simulink model "validationtool"  (R2021b)
settings: Solver=VariableStepAuto  StartTime=0.0  StopTime=2560  FixedStep=0.5  RelTol=1e-3
StopFcn:
  | msg_bs_ctrl.Data=[0];
  | msg_acc_ctrl.Data=[0 0 0 0 0 0 0 0];
undefined symbols (not defined in the file or in its folder): Battery, canChannel, Ts
libraries: canmsglib x28, canlib x4, sharedTrackingLibrary x1
settings Model: Creator=Roland Kummer  LastModifiedBy=Roland Kummer

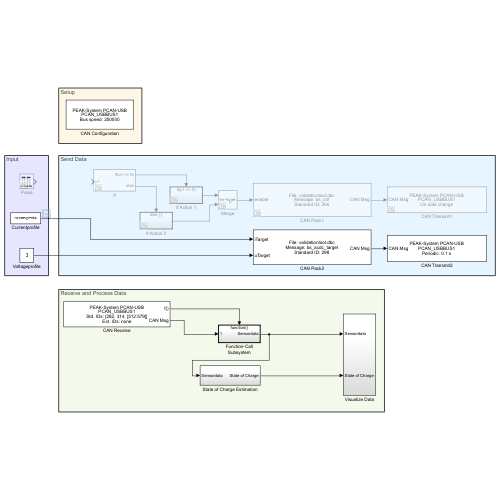
[thumbnail: Simulink's stored preview of the top-level diagram]
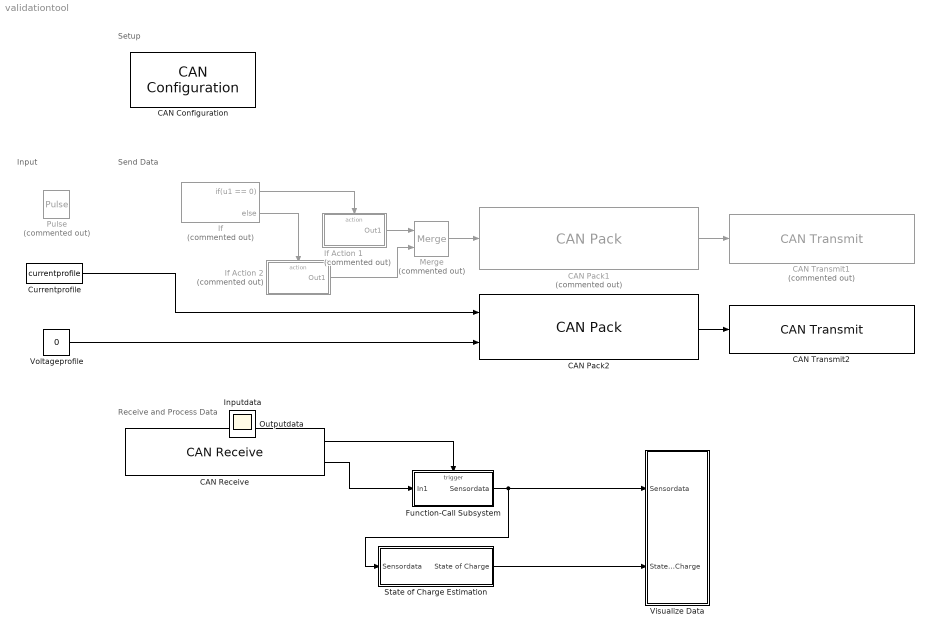
== system validationtool ==
  note: Input
  note: Receive and Process Data
  note: Setup
  note: Send Data
  CAN Configuration : canlib/CAN Configuration  BlockHandle=4.0012  Device=MathWorks Virtual 1 (Channel 1)  DeviceMenu=MathWorks Virtual 1 (Channel 1)  ObjConstructor=canChannel('MathWorks', 'Virtual 1', 1)  BusSpeed=250000  EnableBitParameters=off  AckMode=Normal
      settings: SourceProductBaseCode=VN
  CAN Pack1 : canmsglib/CAN Pack  Commented=on  CANdbFile=C:\Users\Roland Kummer\Documents\Studium\BA-Arbeit\Busmaster\validationtool.dbc  MsgList=bs_ctrl  MsgName=bs_ctrl  MsgIDType=Standard (11-bit identifier)  MsgIdentifier=266  MsgLength=1  Remote=off  ApplyMinMax=off  BusOutput=off  SignalInfo={'enable','0','8','LE','unsigned','Standard','0','1','0','0','2'}
      settings: SourceProductBaseCode=ME,XP,VN  DataFormat=CANdb specified signals
  CAN Pack2 : canmsglib/CAN Pack  CANdbFile=C:\Users\Roland Kummer\Documents\Studium\BA-Arbeit\Busmaster\validationtool.dbc  MsgList=bs_acdc_target  MsgName=bs_acdc_target  MsgIDType=Standard (11-bit identifier)  MsgIdentifier=298  MsgLength=4  Remote=off  ApplyMinMax=off  BusOutput=off  SignalInfo={'iTarget','16','16','LE','unsigned','Standard','0','0.003906','0','0','255.98';'uTarget','0','16','LE','unsigned','Standard','0','0.015625','0','0','0.015625'}
      settings: SourceProductBaseCode=ME,XP,VN  DataFormat=CANdb specified signals
  CAN Receive : canlib/CAN Receive  BlockHandle=7.0012  Device=MathWorks Virtual 1 (Channel 1)  DeviceMenu=MathWorks Virtual 1 (Channel 1)  ObjConstructor=canChannel('MathWorks', 'Virtual 1', 1)  EnableStandardIDsFilter=off  StdIDsCombo=Allow only  StandardIDs=[282, 314, [512:579]]  EnableExtendedIDsFilter=off  ExtIDsCombo=Block all  ExtendedIDs=101  SampleTime=0.1  MsgsPerTimestep=all  InternalFilterUpdateStatus=on  BusOutput=off
      settings: SourceProductBaseCode=VN
  CAN Transmit1 : canlib/CAN Transmit  Commented=on  BlockHandle=8.0012  Device=MathWorks Virtual 1 (Channel 1)  DeviceMenu=MathWorks Virtual 1 (Channel 1)  ObjConstructor=canChannel('MathWorks', 'Virtual 1', 1)  EnableEventTransmit=on  EnablePeriodicTransmit=off  MessagePeriod=0.100
      settings: SourceProductBaseCode=VN
  CAN Transmit2 : canlib/CAN Transmit  BlockHandle=9.0012  Device=MathWorks Virtual 1 (Channel 1)  DeviceMenu=MathWorks Virtual 1 (Channel 1)  ObjConstructor=canChannel('MathWorks', 'Virtual 1', 1)  EnableEventTransmit=off  EnablePeriodicTransmit=on  MessagePeriod=0.100
      settings: SourceProductBaseCode=VN
  Currentprofile : FromWorkspace  VariableName=currentprofile  SampleTime=0.1  Interpolate=off  ZeroCross=off  OutputAfterFinalValue=Setting to zero
  Function-Call Subsystem : Subsystem  TreatAsAtomicUnit=on
  If : If  Commented=on  IfExpression=u1 == 0
  If Action 1 : Subsystem  Commented=on  TreatAsAtomicUnit=on
  If Action 2 : Subsystem  Commented=on  TreatAsAtomicUnit=on
  Merge : Merge  Commented=on
  Pulse : DiscretePulseGenerator  Commented=on  Amplitude=6  Period=1440  PulseWidth=720  PhaseDelay=5
  State of Charge Estimation : Subsystem
  Visualize Data : Subsystem
  Voltageprofile : Constant  Value=0  OutDataTypeStr=double  SampleTime=0.1
  Inputdata : Scope
  Outputdata : Scope
  wires:
  CAN Receive/1 -> Function-Call Subsystem/Trigger
  CAN Receive/2 -> Function-Call Subsystem/1(In1)
  CAN Pack2/1 -> CAN Transmit2/1
  Function-Call Subsystem/1(Sensordata) -> State of Charge Estimation/1(Sensordata), Visualize Data/1(Sensordata)
  State of Charge Estimation/1(State of Charge) -> Visualize Data/2(State of Charge)
  Voltageprofile/1 -> CAN Pack2/2
  CAN Pack1/1 -> CAN Transmit1/1
  If/1 -> If Action 1/Action
  If/2 -> If Action 2/Action
  Merge/1 -> CAN Pack1/1
  If Action 1/1(Out1) -> Merge/1
  If Action 2/1(Out1) -> Merge/2
  Currentprofile/1 -> CAN Pack2/1

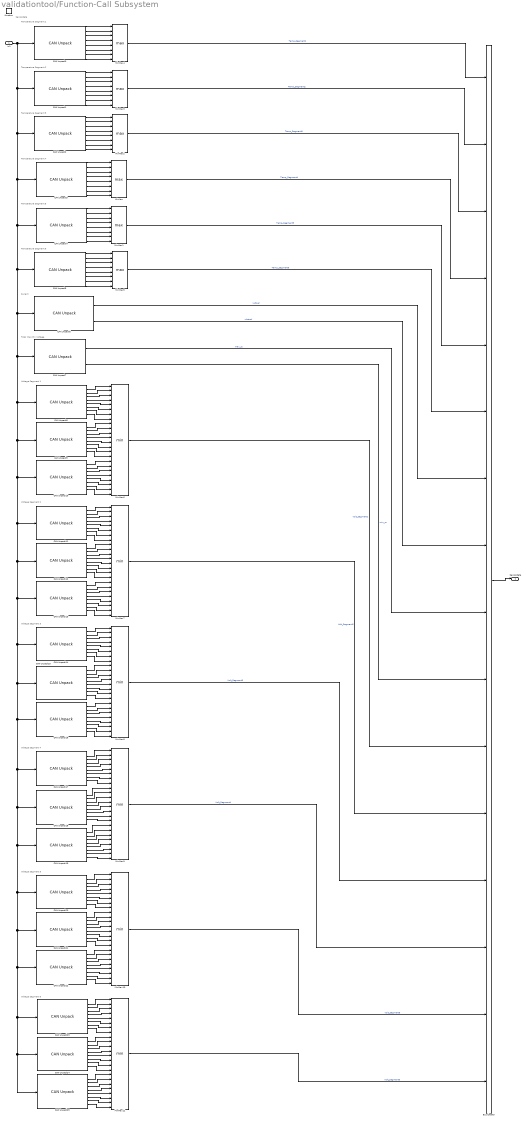
== system validationtool/Function-Call Subsystem ==
  note: Voltage Segment 6
  note: Voltage Segment 2
  note: Voltage Segment 1
  note: Voltage Segment 5
  note: Voltage Segment 4
  note: Voltage Segment 3
  note: Sensordata
  note: Total Max/Min Voltage
  note: Current
  note: Temperature Segment 1
  note: Temperature Segment 2
  note: Temperature Segment 3
  note: Temperature Segment 4
  note: Temperature Segment 6
  note: Temperature Segment 5
  In1 : Inport
  function : TriggerPort  TriggerType=function-call  VariantControl=(inherit)
  Bus Creator : BusCreator  Inputs=16
  CAN Unpack0 : canmsglib/CAN Unpack  CANdbFile=C:\Users\Roland Kummer\Documents\Studium\BA-Arbeit\Busmaster\validationtool.dbc  MsgList=temp1  MsgName=temp1  MsgIDType=Standard (11-bit identifier)  MsgIdentifier=544  MsgLength=8  SignalInfo={'ct1_1','0','8','LE','unsigned','Standard','0','1','0','0','255';'ct1_2','8','8','LE','unsigned','Standard','0','1','0','0','255';'ct1_3','16','8','LE','unsigned','Standard','0','1','0','0','255';'ct1_4','24','8','LE','unsigned','Standard','0','1','0','0','255';'ct1_5','32','8','LE','unsigned','Standard','0','1','0','0','255';'ct1_6','40','8','LE','unsigned','Standard','0','1','0','0','255';'ct1_7','48','8','LE','unsigned','Standard','0','1','0','0','255';'ct1_8','56','1','LE','signed','Standard','0','1','0','0','1'}  IDPort=off  TimestampPort=off  ErrorPort=off  RemotePort=off  LengthPort=off  StatusPort=off  ApplyMinMax=off
      settings: SourceProductBaseCode=ME,XP,VN  DataFormat=CANdb specified signals
  CAN Unpack1 : canmsglib/CAN Unpack  CANdbFile=C:\Users\Roland Kummer\Documents\Studium\BA-Arbeit\Busmaster\validationtool.dbc  MsgList=temp2  MsgName=temp2  MsgIDType=Standard (11-bit identifier)  MsgIdentifier=545  MsgLength=8  SignalInfo={'ct2_1','0','8','LE','unsigned','Standard','0','1','0','0','255';'ct2_2','8','8','LE','unsigned','Standard','0','1','0','0','255';'ct2_3','16','8','LE','unsigned','Standard','0','1','0','0','255';'ct2_4','24','8','LE','unsigned','Standard','0','1','0','0','255';'ct2_5','32','8','LE','unsigned','Standard','0','1','0','0','255';'ct2_6','40','8','LE','unsigned','Standard','0','1','0','0','255';'ct2_7','48','8','LE','unsigned','Standard','0','1','0','0','255';'ct2_8','56','1','LE','signed','Standard','0','1','0','0','1'}  IDPort=off  TimestampPort=off  ErrorPort=off  RemotePort=off  LengthPort=off  StatusPort=off  ApplyMinMax=off
      settings: SourceProductBaseCode=ME,XP,VN  DataFormat=CANdb specified signals
  CAN Unpack10 : canmsglib/CAN Unpack  CANdbFile=C:\Users\Roland Kummer\Documents\Studium\BA-Arbeit\Busmaster\validationtool.dbc  MsgList=cv3  MsgName=cv3  MsgIDType=Standard (11-bit identifier)  MsgIdentifier=514  MsgLength=8  SignalInfo={'cv3_1','0','8','LE','unsigned','Standard','0','0.011765','2','2','5.0001';'cv3_2','8','8','LE','unsigned','Standard','0','0.011765','2','2','5.0001';'cv3_3','16','8','LE','unsigned','Standard','0','0.011765','2','2','5.0001';'cv3_4','24','8','LE','unsigned','Standard','0','0.011765','2','2','5.0001';'cv3_5','32','8','LE','unsigned','Standard','0','0.011765','2','2','5.0001';'cv3_6','40','8','LE','unsigned','Standard','0','0.011765','2','2','5.0001';'cv3_7','48','8','LE','unsigned','Standard','0','0.011765','2','2','5.0001';'cv3_8','56','8','LE','unsigned','Standard','0','0.011765','2','2','5.0001'}  IDPort=off  TimestampPort=off  ErrorPort=off  RemotePort=off  LengthPort=off  StatusPort=off  ApplyMinMax=off
      settings: SourceProductBaseCode=ME,XP,VN  DataFormat=CANdb specified signals
  CAN Unpack11 : canmsglib/CAN Unpack  CANdbFile=C:\Users\Roland Kummer\Documents\Studium\BA-Arbeit\Busmaster\validationtool.dbc  MsgList=cv4  MsgName=cv4  MsgIDType=Standard (11-bit identifier)  MsgIdentifier=515  MsgLength=8  SignalInfo={'cv4_1','0','8','LE','unsigned','Standard','0','0.011765','2','2','5.0001';'cv4_2','8','8','LE','unsigned','Standard','0','0.011765','2','2','5.0001';'cv4_3','16','8','LE','unsigned','Standard','0','0.011765','2','2','5.0001';'cv4_4','24','8','LE','unsigned','Standard','0','0.011765','2','2','5.0001';'cv4_5','32','8','LE','unsigned','Standard','0','0.011765','2','2','5.0001';'cv4_6','40','8','LE','unsigned','Standard','0','0.011765','2','2','5.0001';'cv4_7','48','8','LE','unsigned','Standard','0','0.011765','2','2','5.0001';'cv4_8','56','8','LE','unsigned','Standard','0','0.011765','2','2','5.0001'}  IDPort=off  TimestampPort=off  ErrorPort=off  RemotePort=off  LengthPort=off  StatusPort=off  ApplyMinMax=off
      settings: SourceProductBaseCode=ME,XP,VN  DataFormat=CANdb specified signals
  CAN Unpack12 : canmsglib/CAN Unpack  CANdbFile=C:\Users\Roland Kummer\Documents\Studium\BA-Arbeit\Busmaster\validationtool.dbc  MsgList=cv5  MsgName=cv5  MsgIDType=Standard (11-bit identifier)  MsgIdentifier=516  MsgLength=8  SignalInfo={'cv5_1','0','8','LE','unsigned','Standard','0','0.011765','2','2','5.0001';'cv5_2','8','8','LE','unsigned','Standard','0','0.011765','2','2','5.0001';'cv5_3','16','8','LE','unsigned','Standard','0','0.011765','2','2','5.0001';'cv5_4','24','8','LE','unsigned','Standard','0','0.011765','2','2','5.0001';'cv5_5','32','8','LE','unsigned','Standard','0','0.011765','2','2','5.0001';'cv5_6','40','8','LE','unsigned','Standard','0','0.011765','2','2','5.0001';'cv5_7','48','8','LE','unsigned','Standard','0','0.011765','2','2','5.0001';'cv5_8','56','8','LE','unsigned','Standard','0','0.011765','2','2','5.0001'}  IDPort=off  TimestampPort=off  ErrorPort=off  RemotePort=off  LengthPort=off  StatusPort=off  ApplyMinMax=off
      settings: SourceProductBaseCode=ME,XP,VN  DataFormat=CANdb specified signals
  CAN Unpack13 : canmsglib/CAN Unpack  CANdbFile=C:\Users\Roland Kummer\Documents\Studium\BA-Arbeit\Busmaster\validationtool.dbc  MsgList=cv6  MsgName=cv6  MsgIDType=Standard (11-bit identifier)  MsgIdentifier=517  MsgLength=8  SignalInfo={'cv6_1','0','8','LE','unsigned','Standard','0','0.011765','2','2','5.0001';'cv6_2','8','8','LE','unsigned','Standard','0','0.011765','2','2','5.0001';'cv6_3','16','8','LE','unsigned','Standard','0','0.011765','2','2','5.0001';'cv6_4','24','8','LE','unsigned','Standard','0','0.011765','2','2','5.0001';'cv6_5','32','8','LE','unsigned','Standard','0','0.011765','2','2','5.0001';'cv6_6','40','8','LE','unsigned','Standard','0','0.011765','2','2','5.0001';'cv6_7','48','8','LE','unsigned','Standard','0','0.011765','2','2','5.0001';'cv6_8','56','8','LE','unsigned','Standard','0','0.011765','2','2','5.0001'}  IDPort=off  TimestampPort=off  ErrorPort=off  RemotePort=off  LengthPort=off  StatusPort=off  ApplyMinMax=off
      settings: SourceProductBaseCode=ME,XP,VN  DataFormat=CANdb specified signals
  CAN Unpack14 : canmsglib/CAN Unpack  CANdbFile=C:\Users\Roland Kummer\Documents\Studium\BA-Arbeit\Busmaster\validationtool.dbc  MsgList=cv7  MsgName=cv7  MsgIDType=Standard (11-bit identifier)  MsgIdentifier=518  MsgLength=8  SignalInfo={'cv7_1','0','8','LE','unsigned','Standard','0','0.011765','2','2','5.0001';'cv7_2','8','8','LE','unsigned','Standard','0','0.011765','2','2','5.0001';'cv7_3','16','8','LE','unsigned','Standard','0','0.011765','2','2','5.0001';'cv7_4','24','8','LE','unsigned','Standard','0','0.011765','2','2','5.0001';'cv7_5','32','8','LE','unsigned','Standard','0','0.011765','2','2','5.0001';'cv7_6','40','8','LE','unsigned','Standard','0','0.011765','2','2','5.0001';'cv7_7','48','8','LE','unsigned','Standard','0','0.011765','2','2','5.0001';'cv7_8','56','8','LE','unsigned','Standard','0','0.011765','2','2','5.0001'}  IDPort=off  TimestampPort=off  ErrorPort=off  RemotePort=off  LengthPort=off  StatusPort=off  ApplyMinMax=off
      settings: SourceProductBaseCode=ME,XP,VN  DataFormat=CANdb specified signals
  CAN Unpack15 : canmsglib/CAN Unpack  CANdbFile=C:\Users\Roland Kummer\Documents\Studium\BA-Arbeit\Busmaster\validationtool.dbc  MsgList=cv8  MsgName=cv8  MsgIDType=Standard (11-bit identifier)  MsgIdentifier=519  MsgLength=8  SignalInfo={'cv8_1','0','8','LE','unsigned','Standard','0','0.011765','2','2','5.0001';'cv8_2','8','8','LE','unsigned','Standard','0','0.011765','2','2','5.0001';'cv8_3','16','8','LE','unsigned','Standard','0','0.011765','2','2','5.0001';'cv8_4','24','8','LE','unsigned','Standard','0','0.011765','2','2','5.0001';'cv8_5','32','8','LE','unsigned','Standard','0','0.011765','2','2','5.0001';'cv8_6','40','8','LE','unsigned','Standard','0','0.011765','2','2','5.0001';'cv8_7','48','8','LE','unsigned','Standard','0','0.011765','2','2','5.0001';'cv8_8','56','8','LE','unsigned','Standard','0','0.011765','2','2','5.0001'}  IDPort=off  TimestampPort=off  ErrorPort=off  RemotePort=off  LengthPort=off  StatusPort=off  ApplyMinMax=off
      settings: SourceProductBaseCode=ME,XP,VN  DataFormat=CANdb specified signals
  CAN Unpack16 : canmsglib/CAN Unpack  CANdbFile=C:\Users\Roland Kummer\Documents\Studium\BA-Arbeit\Busmaster\validationtool.dbc  MsgList=cv9  MsgName=cv9  MsgIDType=Standard (11-bit identifier)  MsgIdentifier=520  MsgLength=8  SignalInfo={'cv9_1','0','8','LE','unsigned','Standard','0','0.011765','2','2','5.0001';'cv9_2','8','8','LE','unsigned','Standard','0','0.011765','2','2','5.0001';'cv9_3','16','8','LE','unsigned','Standard','0','0.011765','2','2','5.0001';'cv9_4','24','8','LE','unsigned','Standard','0','0.011765','2','2','5.0001';'cv9_5','32','8','LE','unsigned','Standard','0','0.011765','2','2','5.0001';'cv9_6','40','8','LE','unsigned','Standard','0','0.011765','2','2','5.0001';'cv9_7','48','8','LE','unsigned','Standard','0','0.011765','2','2','5.0001';'cv9_8','56','8','LE','unsigned','Standard','0','0.011765','2','2','5.0001'}  IDPort=off  TimestampPort=off  ErrorPort=off  RemotePort=off  LengthPort=off  StatusPort=off  ApplyMinMax=off
      settings: SourceProductBaseCode=ME,XP,VN  DataFormat=CANdb specified signals
  CAN Unpack17 : canmsglib/CAN Unpack  CANdbFile=C:\Users\Roland Kummer\Documents\Studium\BA-Arbeit\Busmaster\validationtool.dbc  MsgList=cv10  MsgName=cv10  MsgIDType=Standard (11-bit identifier)  MsgIdentifier=521  MsgLength=8  SignalInfo={'cv10_1','0','8','LE','unsigned','Standard','0','0.011765','2','2','5.0001';'cv10_2','8','8','LE','unsigned','Standard','0','0.011765','2','2','5.0001';'cv10_3','16','8','LE','unsigned','Standard','0','0.011765','2','2','5.0001';'cv10_4','24','8','LE','unsigned','Standard','0','0.011765','2','2','5.0001';'cv10_5','32','8','LE','unsigned','Standard','0','0.011765','2','2','5.0001';'cv10_6','40','8','LE','unsigned','Standard','0','0.011765','2','2','5.0001';'cv10_7','48','8','LE','unsigned','Standard','0','0.011765','2','2','5.0001';'cv10_8','56','8','LE','unsigned','Standard','0','0.011765','2','2','5.0001'}  IDPort=off  TimestampPort=off  ErrorPort=off  RemotePort=off  LengthPort=off  StatusPort=off  ApplyMinMax=off
      settings: SourceProductBaseCode=ME,XP,VN  DataFormat=CANdb specified signals
  CAN Unpack18 : canmsglib/CAN Unpack  CANdbFile=C:\Users\Roland Kummer\Documents\Studium\BA-Arbeit\Busmaster\validationtool.dbc  MsgList=cv11  MsgName=cv11  MsgIDType=Standard (11-bit identifier)  MsgIdentifier=522  MsgLength=8  SignalInfo={'cv11_1','0','8','LE','unsigned','Standard','0','0.011765','2','2','5.0001';'cv11_2','8','8','LE','unsigned','Standard','0','0.011765','2','2','5.0001';'cv11_3','16','8','LE','unsigned','Standard','0','0.011765','2','2','5.0001';'cv11_4','24','8','LE','unsigned','Standard','0','0.011765','2','2','5.0001';'cv11_5','32','8','LE','unsigned','Standard','0','0.011765','2','2','5.0001';'cv11_6','40','8','LE','unsigned','Standard','0','0.011765','2','2','5.0001';'cv11_7','48','8','LE','unsigned','Standard','0','0.011765','2','2','5.0001';'cv11_8','56','8','LE','unsigned','Standard','0','0.011765','2','2','5.0001'}  IDPort=off  TimestampPort=off  ErrorPort=off  RemotePort=off  LengthPort=off  StatusPort=off  ApplyMinMax=off
      settings: SourceProductBaseCode=ME,XP,VN  DataFormat=CANdb specified signals
  CAN Unpack19 : canmsglib/CAN Unpack  CANdbFile=C:\Users\Roland Kummer\Documents\Studium\BA-Arbeit\Busmaster\validationtool.dbc  MsgList=cv12  MsgName=cv12  MsgIDType=Standard (11-bit identifier)  MsgIdentifier=523  MsgLength=8  SignalInfo={'cv12_1','0','8','LE','unsigned','Standard','0','0.011765','2','2','5.0001';'cv12_2','8','8','LE','unsigned','Standard','0','0.011765','2','2','5.0001';'cv12_3','16','8','LE','unsigned','Standard','0','0.011765','2','2','5.0001';'cv12_4','24','8','LE','unsigned','Standard','0','0.011765','2','2','5.0001';'cv12_5','32','8','LE','unsigned','Standard','0','0.011765','2','2','5.0001';'cv12_6','40','8','LE','unsigned','Standard','0','0.011765','2','2','5.0001';'cv12_7','48','8','LE','unsigned','Standard','0','0.011765','2','2','5.0001';'cv12_8','56','8','LE','unsigned','Standard','0','0.011765','2','2','5.0001'}  IDPort=off  TimestampPort=off  ErrorPort=off  RemotePort=off  LengthPort=off  StatusPort=off  ApplyMinMax=off
      settings: SourceProductBaseCode=ME,XP,VN  DataFormat=CANdb specified signals
  CAN Unpack2 : canmsglib/CAN Unpack  CANdbFile=C:\Users\Roland Kummer\Documents\Studium\BA-Arbeit\Busmaster\validationtool.dbc  MsgList=temp3  MsgName=temp3  MsgIDType=Standard (11-bit identifier)  MsgIdentifier=546  MsgLength=8  SignalInfo={'ct3_1','0','8','LE','unsigned','Standard','0','1','0','0','255';'ct3_2','8','8','LE','unsigned','Standard','0','1','0','0','255';'ct3_3','16','8','LE','unsigned','Standard','0','1','0','0','255';'ct3_4','24','8','LE','unsigned','Standard','0','1','0','0','255';'ct3_5','32','8','LE','unsigned','Standard','0','1','0','0','255';'ct3_6','40','8','LE','unsigned','Standard','0','1','0','0','255';'ct3_7','48','8','LE','unsigned','Standard','0','1','0','0','255';'ct3_8','56','1','LE','signed','Standard','0','1','0','0','1'}  IDPort=off  TimestampPort=off  ErrorPort=off  RemotePort=off  LengthPort=off  StatusPort=off  ApplyMinMax=off
      settings: SourceProductBaseCode=ME,XP,VN  DataFormat=CANdb specified signals
  CAN Unpack20 : canmsglib/CAN Unpack  CANdbFile=C:\Users\Roland Kummer\Documents\Studium\BA-Arbeit\Busmaster\validationtool.dbc  MsgList=cv13  MsgName=cv13  MsgIDType=Standard (11-bit identifier)  MsgIdentifier=524  MsgLength=8  SignalInfo={'cv13_1','0','8','LE','unsigned','Standard','0','0.011765','2','2','5.0001';'cv13_2','8','8','LE','unsigned','Standard','0','0.011765','2','2','5.0001';'cv13_3','16','8','LE','unsigned','Standard','0','0.011765','2','2','5.0001';'cv13_4','24','8','LE','unsigned','Standard','0','0.011765','2','2','5.0001';'cv13_5','32','8','LE','unsigned','Standard','0','0.011765','2','2','5.0001';'cv13_6','40','8','LE','unsigned','Standard','0','0.011765','2','2','5.0001';'cv13_7','48','8','LE','unsigned','Standard','0','0.011765','2','2','5.0001';'cv13_8','56','8','LE','unsigned','Standard','0','0.011765','2','2','5.0001'}  IDPort=off  TimestampPort=off  ErrorPort=off  RemotePort=off  LengthPort=off  StatusPort=off  ApplyMinMax=off
      settings: SourceProductBaseCode=ME,XP,VN  DataFormat=CANdb specified signals
  CAN Unpack21 : canmsglib/CAN Unpack  CANdbFile=C:\Users\Roland Kummer\Documents\Studium\BA-Arbeit\Busmaster\validationtool.dbc  MsgList=cv14  MsgName=cv14  MsgIDType=Standard (11-bit identifier)  MsgIdentifier=525  MsgLength=8  SignalInfo={'cv14_1','0','8','LE','unsigned','Standard','0','0.011765','2','2','5.0001';'cv14_2','8','8','LE','unsigned','Standard','0','0.011765','2','2','5.0001';'cv14_3','16','8','LE','unsigned','Standard','0','0.011765','2','2','5.0001';'cv14_4','24','8','LE','unsigned','Standard','0','0.011765','2','2','5.0001';'cv14_5','32','8','LE','unsigned','Standard','0','0.011765','2','2','5.0001';'cv14_6','40','8','LE','unsigned','Standard','0','0.011765','2','2','5.0001';'cv14_7','48','8','LE','unsigned','Standard','0','0.011765','2','2','5.0001';'cv14_8','56','8','LE','unsigned','Standard','0','0.011765','2','2','5.0001'}  IDPort=off  TimestampPort=off  ErrorPort=off  RemotePort=off  LengthPort=off  StatusPort=off  ApplyMinMax=off
      settings: SourceProductBaseCode=ME,XP,VN  DataFormat=CANdb specified signals
  CAN Unpack22 : canmsglib/CAN Unpack  CANdbFile=C:\Users\Roland Kummer\Documents\Studium\BA-Arbeit\Busmaster\validationtool.dbc  MsgList=cv15  MsgName=cv15  MsgIDType=Standard (11-bit identifier)  MsgIdentifier=526  MsgLength=8  SignalInfo={'cv15_1','0','8','LE','unsigned','Standard','0','0.011765','2','2','5.0001';'cv15_2','8','8','LE','unsigned','Standard','0','0.011765','2','2','5.0001';'cv15_3','16','8','LE','unsigned','Standard','0','0.011765','2','2','5.0001';'cv15_4','24','8','LE','unsigned','Standard','0','0.011765','2','2','5.0001';'cv15_5','32','8','LE','unsigned','Standard','0','0.011765','2','2','5.0001';'cv15_6','40','8','LE','unsigned','Standard','0','0.011765','2','2','5.0001';'cv15_7','48','8','LE','unsigned','Standard','0','0.011765','2','2','5.0001';'cv15_8','56','8','LE','unsigned','Standard','0','0.011765','2','2','5.0001'}  IDPort=off  TimestampPort=off  ErrorPort=off  RemotePort=off  LengthPort=off  StatusPort=off  ApplyMinMax=off
      settings: SourceProductBaseCode=ME,XP,VN  DataFormat=CANdb specified signals
  CAN Unpack23 : canmsglib/CAN Unpack  CANdbFile=C:\Users\Roland Kummer\Documents\Studium\BA-Arbeit\Busmaster\validationtool.dbc  MsgList=cv16  MsgName=cv16  MsgIDType=Standard (11-bit identifier)  MsgIdentifier=527  MsgLength=8  SignalInfo={'cv16_1','0','8','LE','unsigned','Standard','0','0.011765','2','2','5.0001';'cv16_2','8','8','LE','unsigned','Standard','0','0.011765','2','2','5.0001';'cv16_3','16','8','LE','unsigned','Standard','0','0.011765','2','2','5.0001';'cv16_4','24','8','LE','unsigned','Standard','0','0.011765','2','2','5.0001';'cv16_5','32','8','LE','unsigned','Standard','0','0.011765','2','2','5.0001';'cv16_6','40','8','LE','unsigned','Standard','0','0.011765','2','2','5.0001';'cv16_7','48','8','LE','unsigned','Standard','0','0.011765','2','2','5.0001';'cv16_8','56','8','LE','unsigned','Standard','0','0.011765','2','2','5.0001'}  IDPort=off  TimestampPort=off  ErrorPort=off  RemotePort=off  LengthPort=off  StatusPort=off  ApplyMinMax=off
      settings: SourceProductBaseCode=ME,XP,VN  DataFormat=CANdb specified signals
  CAN Unpack24 : canmsglib/CAN Unpack  CANdbFile=C:\Users\Roland Kummer\Documents\Studium\BA-Arbeit\Busmaster\validationtool.dbc  MsgList=cv17  MsgName=cv17  MsgIDType=Standard (11-bit identifier)  MsgIdentifier=528  MsgLength=8  SignalInfo={'cv17_1','0','8','LE','unsigned','Standard','0','0.011765','2','2','5.0001';'cv17_2','8','8','LE','unsigned','Standard','0','0.011765','2','2','5.0001';'cv17_3','16','8','LE','unsigned','Standard','0','0.011765','2','2','5.0001';'cv17_4','24','8','LE','unsigned','Standard','0','0.011765','2','2','5.0001';'cv17_5','32','8','LE','unsigned','Standard','0','0.011765','2','2','5.0001';'cv17_6','40','8','LE','unsigned','Standard','0','0.011765','2','2','5.0001';'cv17_7','48','8','LE','unsigned','Standard','0','0.011765','2','2','5.0001';'cv17_8','56','8','LE','unsigned','Standard','0','0.011765','2','2','5.0001'}  IDPort=off  TimestampPort=off  ErrorPort=off  RemotePort=off  LengthPort=off  StatusPort=off  ApplyMinMax=off
      settings: SourceProductBaseCode=ME,XP,VN  DataFormat=CANdb specified signals
  CAN Unpack25 : canmsglib/CAN Unpack  CANdbFile=C:\Users\Roland Kummer\Documents\Studium\BA-Arbeit\Busmaster\validationtool.dbc  MsgList=cv18  MsgName=cv18  MsgIDType=Standard (11-bit identifier)  MsgIdentifier=529  MsgLength=8  SignalInfo={'cv18_1','0','8','LE','unsigned','Standard','0','0.011765','2','2','5.0001';'cv18_2','8','8','LE','unsigned','Standard','0','0.011765','2','2','5.0001';'cv18_3','16','8','LE','unsigned','Standard','0','0.011765','2','2','5.0001';'cv18_4','24','8','LE','unsigned','Standard','0','0.011765','2','2','5.0001';'cv18_5','32','8','LE','unsigned','Standard','0','0.011765','2','2','5.0001';'cv18_6','40','8','LE','unsigned','Standard','0','0.011765','2','2','5.0001';'cv18_7','48','8','LE','unsigned','Standard','0','0.011765','2','2','5.0001';'cv18_8','56','8','LE','unsigned','Standard','0','0.011765','2','2','5.0001'}  IDPort=off  TimestampPort=off  ErrorPort=off  RemotePort=off  LengthPort=off  StatusPort=off  ApplyMinMax=off
      settings: SourceProductBaseCode=ME,XP,VN  DataFormat=CANdb specified signals
  CAN Unpack3 : canmsglib/CAN Unpack  CANdbFile=C:\Users\Roland Kummer\Documents\Studium\BA-Arbeit\Busmaster\validationtool.dbc  MsgList=temp4  MsgName=temp4  MsgIDType=Standard (11-bit identifier)  MsgIdentifier=547  MsgLength=8  SignalInfo={'ct4_1','0','8','LE','unsigned','Standard','0','1','0','0','255';'ct4_2','8','8','LE','unsigned','Standard','0','1','0','0','255';'ct4_3','16','8','LE','unsigned','Standard','0','1','0','0','255';'ct4_4','24','8','LE','unsigned','Standard','0','1','0','0','255';'ct4_5','32','8','LE','unsigned','Standard','0','1','0','0','255';'ct4_6','40','8','LE','unsigned','Standard','0','1','0','0','255';'ct4_7','48','8','LE','unsigned','Standard','0','1','0','0','255';'ct4_8','56','1','LE','signed','Standard','0','1','0','0','1'}  IDPort=off  TimestampPort=off  ErrorPort=off  RemotePort=off  LengthPort=off  StatusPort=off  ApplyMinMax=off
      settings: SourceProductBaseCode=ME,XP,VN  DataFormat=CANdb specified signals
  CAN Unpack4 : canmsglib/CAN Unpack  CANdbFile=C:\Users\Roland Kummer\Documents\Studium\BA-Arbeit\Busmaster\validationtool.dbc  MsgList=temp5  MsgName=temp5  MsgIDType=Standard (11-bit identifier)  MsgIdentifier=548  MsgLength=8  SignalInfo={'ct5_1','0','8','LE','unsigned','Standard','0','1','0','0','255';'ct5_2','8','8','LE','unsigned','Standard','0','1','0','0','255';'ct5_3','16','8','LE','unsigned','Standard','0','1','0','0','255';'ct5_4','24','8','LE','unsigned','Standard','0','1','0','0','255';'ct5_5','32','8','LE','unsigned','Standard','0','1','0','0','255';'ct5_6','40','8','LE','unsigned','Standard','0','1','0','0','255';'ct5_7','48','8','LE','unsigned','Standard','0','1','0','0','255';'ct5_8','56','1','LE','signed','Standard','0','1','0','0','1'}  IDPort=off  TimestampPort=off  ErrorPort=off  RemotePort=off  LengthPort=off  StatusPort=off  ApplyMinMax=off
      settings: SourceProductBaseCode=ME,XP,VN  DataFormat=CANdb specified signals
  CAN Unpack5 : canmsglib/CAN Unpack  CANdbFile=C:\Users\Roland Kummer\Documents\Studium\BA-Arbeit\Busmaster\validationtool.dbc  MsgList=temp6  MsgName=temp6  MsgIDType=Standard (11-bit identifier)  MsgIdentifier=549  MsgLength=8  SignalInfo={'ct6_1','0','8','LE','unsigned','Standard','0','1','0','0','255';'ct6_2','8','8','LE','unsigned','Standard','0','1','0','0','255';'ct6_3','16','8','LE','unsigned','Standard','0','1','0','0','255';'ct6_4','24','8','LE','unsigned','Standard','0','1','0','0','255';'ct6_5','32','8','LE','unsigned','Standard','0','1','0','0','255';'ct6_6','40','8','LE','unsigned','Standard','0','1','0','0','255';'ct6_7','48','8','LE','unsigned','Standard','0','1','0','0','255';'ct6_8','56','1','LE','signed','Standard','0','1','0','0','1'}  IDPort=off  TimestampPort=off  ErrorPort=off  RemotePort=off  LengthPort=off  StatusPort=off  ApplyMinMax=off
      settings: SourceProductBaseCode=ME,XP,VN  DataFormat=CANdb specified signals
  CAN Unpack6 : canmsglib/CAN Unpack  CANdbFile=C:\Users\Roland Kummer\Documents\Studium\BA-Arbeit\Busmaster\validationtool.dbc  MsgList=bs_acdc_actual  MsgName=bs_acdc_actual  MsgIDType=Standard (11-bit identifier)  MsgIdentifier=314  MsgLength=4  SignalInfo={'iActual','16','16','LE','unsigned','Standard','0','0.003906','0','0','255.98';'uActual','0','16','LE','unsigned','Standard','0','0.015625','0','0','1023.98'}  IDPort=off  TimestampPort=off  ErrorPort=off  RemotePort=off  LengthPort=off  StatusPort=off  ApplyMinMax=off
      settings: SourceProductBaseCode=ME,XP,VN  DataFormat=CANdb specified signals
  CAN Unpack7 : canmsglib/CAN Unpack  CANdbFile=C:\Users\Roland Kummer\Documents\Studium\BA-Arbeit\Busmaster\validationtool.dbc  MsgList=accu_signal_1  MsgName=accu_signal_1  MsgIDType=Standard (11-bit identifier)  MsgIdentifier=576  MsgLength=8  SignalInfo={'max_cv','8','16','BE','unsigned','Standard','0','0.0001','0','0','6.5535';'min_cv','24','16','BE','unsigned','Standard','0','0.0001','0','0','6.5535'}  IDPort=off  TimestampPort=off  ErrorPort=off  RemotePort=off  LengthPort=off  StatusPort=off  ApplyMinMax=off
      settings: SourceProductBaseCode=ME,XP,VN  DataFormat=CANdb specified signals
  CAN Unpack8 : canmsglib/CAN Unpack  CANdbFile=C:\Users\Roland Kummer\Documents\Studium\BA-Arbeit\Busmaster\validationtool.dbc  MsgList=cv1  MsgName=cv1  MsgIDType=Standard (11-bit identifier)  MsgIdentifier=512  MsgLength=8  SignalInfo={'cv1_1','0','8','LE','unsigned','Standard','0','0.011765','2','2','5.0001';'cv1_2','8','8','LE','unsigned','Standard','0','0.011765','2','2','5.0001';'cv1_3','16','8','LE','unsigned','Standard','0','0.011765','2','2','5.0001';'cv1_4','24','8','LE','unsigned','Standard','0','0.011765','2','2','5.0001';'cv1_5','32','8','LE','unsigned','Standard','0','0.011765','2','2','5.0001';'cv1_6','40','8','LE','unsigned','Standard','0','0.011765','2','2','5.0001';'cv1_7','48','8','LE','unsigned','Standard','0','0.011765','2','2','5.0001';'cv1_8','56','8','LE','unsigned','Standard','0','0.011765','2','2','5.0001'}  IDPort=off  TimestampPort=off  ErrorPort=off  RemotePort=off  LengthPort=off  StatusPort=off  ApplyMinMax=off
      settings: SourceProductBaseCode=ME,XP,VN  DataFormat=CANdb specified signals
  CAN Unpack9 : canmsglib/CAN Unpack  CANdbFile=C:\Users\Roland Kummer\Documents\Studium\BA-Arbeit\Busmaster\validationtool.dbc  MsgList=cv2  MsgName=cv2  MsgIDType=Standard (11-bit identifier)  MsgIdentifier=513  MsgLength=8  SignalInfo={'cv2_1','0','8','LE','unsigned','Standard','0','0.011765','2','2','5.0001';'cv2_2','8','8','LE','unsigned','Standard','0','0.011765','2','2','5.0001';'cv2_3','16','8','LE','unsigned','Standard','0','0.011765','2','2','5.0001';'cv2_4','24','8','LE','unsigned','Standard','0','0.011765','2','2','5.0001';'cv2_5','32','8','LE','unsigned','Standard','0','0.011765','2','2','5.0001';'cv2_6','40','8','LE','unsigned','Standard','0','0.011765','2','2','5.0001';'cv2_7','48','8','LE','unsigned','Standard','0','0.011765','2','2','5.0001';'cv2_8','56','8','LE','unsigned','Standard','0','0.011765','2','2','5.0001'}  IDPort=off  TimestampPort=off  ErrorPort=off  RemotePort=off  LengthPort=off  StatusPort=off  ApplyMinMax=off
      settings: SourceProductBaseCode=ME,XP,VN  DataFormat=CANdb specified signals
  MinMax{,1..5} (6 alike) : MinMax  Function=max  Inputs=8
  MinMax{6..11} (6 alike) : MinMax  Inputs=24
  Sensordata : Outport
  wires:
  In1/1 -> CAN Unpack6/1, CAN Unpack7/1, CAN Unpack8/1, CAN Unpack9/1, CAN Unpack10/1, CAN Unpack11/1, CAN Unpack12/1, CAN Unpack13/1, CAN Unpack14/1, CAN Unpack15/1, CAN Unpack16/1, CAN Unpack17/1, CAN Unpack18/1, CAN Unpack19/1, CAN Unpack20/1, CAN Unpack21/1, CAN Unpack22/1, CAN Unpack23/1, CAN Unpack24/1, CAN Unpack25/1, CAN Unpack5/1, CAN Unpack4/1, CAN Unpack3/1, CAN Unpack2/1, CAN Unpack1/1, CAN Unpack0/1
  CAN Unpack13/8 -> MinMax7/24
  CAN Unpack8/1 -> MinMax6/1
  CAN Unpack8/2 -> MinMax6/2
  CAN Unpack8/3 -> MinMax6/3
  CAN Unpack8/5 -> MinMax6/5
  CAN Unpack8/6 -> MinMax6/6
  CAN Unpack8/7 -> MinMax6/7
  CAN Unpack8/8 -> MinMax6/8
  CAN Unpack9/1 -> MinMax6/9
  CAN Unpack9/2 -> MinMax6/10
  CAN Unpack9/3 -> MinMax6/11
  CAN Unpack9/4 -> MinMax6/12
  CAN Unpack9/5 -> MinMax6/13
  CAN Unpack9/6 -> MinMax6/14
  CAN Unpack9/7 -> MinMax6/15
  CAN Unpack9/8 -> MinMax6/16
  CAN Unpack10/1 -> MinMax6/17
  CAN Unpack10/2 -> MinMax6/18
  CAN Unpack10/3 -> MinMax6/19
  CAN Unpack10/4 -> MinMax6/20
  CAN Unpack10/5 -> MinMax6/21
  CAN Unpack10/6 -> MinMax6/22
  CAN Unpack10/7 -> MinMax6/23
  CAN Unpack10/8 -> MinMax6/24
  CAN Unpack11/1 -> MinMax7/1
  CAN Unpack11/2 -> MinMax7/2
  CAN Unpack11/3 -> MinMax7/3
  CAN Unpack11/4 -> MinMax7/4
  CAN Unpack11/5 -> MinMax7/5
  CAN Unpack11/6 -> MinMax7/6
  CAN Unpack11/7 -> MinMax7/7
  CAN Unpack11/8 -> MinMax7/8
  CAN Unpack12/1 -> MinMax7/9
  CAN Unpack12/2 -> MinMax7/10
  CAN Unpack12/3 -> MinMax7/11
  CAN Unpack12/4 -> MinMax7/12
  CAN Unpack12/5 -> MinMax7/13
  CAN Unpack12/6 -> MinMax7/14
  CAN Unpack12/7 -> MinMax7/15
  CAN Unpack12/8 -> MinMax7/16
  CAN Unpack13/1 -> MinMax7/17
  CAN Unpack13/2 -> MinMax7/18
  CAN Unpack13/3 -> MinMax7/19
  CAN Unpack13/4 -> MinMax7/20
  CAN Unpack13/5 -> MinMax7/21
  CAN Unpack13/6 -> MinMax7/22
  CAN Unpack13/7 -> MinMax7/23
  CAN Unpack14/1 -> MinMax8/1
  CAN Unpack14/2 -> MinMax8/2
  CAN Unpack14/3 -> MinMax8/3
  CAN Unpack14/4 -> MinMax8/4
  CAN Unpack14/5 -> MinMax8/5
  CAN Unpack14/6 -> MinMax8/6
  CAN Unpack14/7 -> MinMax8/7
  CAN Unpack14/8 -> MinMax8/8
  CAN Unpack15/1 -> MinMax8/9
  CAN Unpack15/2 -> MinMax8/10
  CAN Unpack15/3 -> MinMax8/11
  CAN Unpack15/4 -> MinMax8/12
  CAN Unpack15/5 -> MinMax8/13
  CAN Unpack15/6 -> MinMax8/14
  CAN Unpack15/7 -> MinMax8/15
  CAN Unpack15/8 -> MinMax8/16
  CAN Unpack16/1 -> MinMax8/17
  CAN Unpack16/2 -> MinMax8/18
  CAN Unpack16/3 -> MinMax8/19
  CAN Unpack16/4 -> MinMax8/20
  CAN Unpack16/5 -> MinMax8/21
  CAN Unpack16/6 -> MinMax8/22
  CAN Unpack16/7 -> MinMax8/23
  CAN Unpack16/8 -> MinMax8/24
  CAN Unpack17/1 -> MinMax9/1
  CAN Unpack17/2 -> MinMax9/2
  CAN Unpack17/3 -> MinMax9/3
  CAN Unpack17/4 -> MinMax9/4
  CAN Unpack17/5 -> MinMax9/5
  CAN Unpack17/6 -> MinMax9/6
  CAN Unpack17/7 -> MinMax9/7
  CAN Unpack17/8 -> MinMax9/8
  CAN Unpack18/1 -> MinMax9/9
  CAN Unpack18/2 -> MinMax9/10
  CAN Unpack18/3 -> MinMax9/11
  CAN Unpack18/4 -> MinMax9/12
  CAN Unpack18/5 -> MinMax9/13
  CAN Unpack18/6 -> MinMax9/14
  CAN Unpack18/7 -> MinMax9/15
  CAN Unpack18/8 -> MinMax9/16
  CAN Unpack19/1 -> MinMax9/17
  CAN Unpack19/2 -> MinMax9/18
  CAN Unpack19/3 -> MinMax9/19
  CAN Unpack19/4 -> MinMax9/20
  CAN Unpack19/5 -> MinMax9/21
  CAN Unpack19/6 -> MinMax9/22
  CAN Unpack19/7 -> MinMax9/23
  CAN Unpack19/8 -> MinMax9/24
  CAN Unpack20/1 -> MinMax10/1
  CAN Unpack20/2 -> MinMax10/2
  CAN Unpack20/3 -> MinMax10/3
  CAN Unpack20/4 -> MinMax10/4
  CAN Unpack20/5 -> MinMax10/5
  CAN Unpack20/6 -> MinMax10/6
  CAN Unpack20/7 -> MinMax10/7
  CAN Unpack20/8 -> MinMax10/8
  CAN Unpack21/1 -> MinMax10/9
  CAN Unpack21/2 -> MinMax10/10
  CAN Unpack21/3 -> MinMax10/11
  CAN Unpack21/4 -> MinMax10/12
  CAN Unpack21/5 -> MinMax10/13
  CAN Unpack21/6 -> MinMax10/14
  CAN Unpack21/7 -> MinMax10/15
  CAN Unpack21/8 -> MinMax10/16
  CAN Unpack22/1 -> MinMax10/17
  CAN Unpack22/2 -> MinMax10/18
  CAN Unpack22/3 -> MinMax10/19
  CAN Unpack22/4 -> MinMax10/20
  CAN Unpack22/5 -> MinMax10/21
  CAN Unpack22/6 -> MinMax10/22
  CAN Unpack22/7 -> MinMax10/23
  CAN Unpack22/8 -> MinMax10/24
  CAN Unpack23/1 -> MinMax11/1
  CAN Unpack23/2 -> MinMax11/2
  CAN Unpack23/3 -> MinMax11/3
  CAN Unpack23/4 -> MinMax11/4
  CAN Unpack23/5 -> MinMax11/5
  CAN Unpack23/6 -> MinMax11/6
  CAN Unpack23/7 -> MinMax11/7
  CAN Unpack23/8 -> MinMax11/8
  CAN Unpack24/1 -> MinMax11/9
  CAN Unpack24/2 -> MinMax11/10
  CAN Unpack24/3 -> MinMax11/11
  CAN Unpack24/4 -> MinMax11/12
  CAN Unpack24/5 -> MinMax11/13
  CAN Unpack24/6 -> MinMax11/14
  CAN Unpack24/7 -> MinMax11/15
  CAN Unpack24/8 -> MinMax11/16
  CAN Unpack25/1 -> MinMax11/17
  CAN Unpack25/2 -> MinMax11/18
  CAN Unpack25/3 -> MinMax11/19
  CAN Unpack25/4 -> MinMax11/20
  CAN Unpack25/5 -> MinMax11/21
  CAN Unpack25/6 -> MinMax11/22
  CAN Unpack25/7 -> MinMax11/23
  CAN Unpack25/8 -> MinMax11/24
  MinMax4/1 -> Bus Creator/1  "Temp_Segment1"
  MinMax3/1 -> Bus Creator/2  "Temp_Segment2"
  MinMax2/1 -> Bus Creator/3  "Temp_Segment3"
  MinMax/1 -> Bus Creator/4  "Temp_Segment4"
  MinMax5/1 -> Bus Creator/6  "Temp_Segment6"
  CAN Unpack7/1 -> Bus Creator/9  "max_cv"
  CAN Unpack7/2 -> Bus Creator/10  "min_cv"
  MinMax1/1 -> Bus Creator/5  "Temp_Segment5"
  Bus Creator/1 -> Sensordata/1
  MinMax6/1 -> Bus Creator/11  "Volt_Segment1"
  MinMax7/1 -> Bus Creator/12  "Volt_Segment2"
  MinMax8/1 -> Bus Creator/13  "Volt_Segment3"
  MinMax9/1 -> Bus Creator/14  "Volt_Segment4"
  MinMax10/1 -> Bus Creator/15  "Volt_Segment5"
  MinMax11/1 -> Bus Creator/16  "Volt_Segment6"
  CAN Unpack6/1 -> Bus Creator/7  "iActual"
  CAN Unpack6/2 -> Bus Creator/8  "uActual"
  CAN Unpack8/4 -> MinMax6/4
  CAN Unpack0/1 -> MinMax4/1
  CAN Unpack0/2 -> MinMax4/2
  CAN Unpack0/3 -> MinMax4/3
  CAN Unpack0/4 -> MinMax4/4
  CAN Unpack0/5 -> MinMax4/5
  CAN Unpack0/6 -> MinMax4/6
  CAN Unpack0/7 -> MinMax4/7
  CAN Unpack0/8 -> MinMax4/8
  CAN Unpack1/1 -> MinMax3/1
  CAN Unpack1/2 -> MinMax3/2
  CAN Unpack1/3 -> MinMax3/3
  CAN Unpack1/4 -> MinMax3/4
  CAN Unpack1/5 -> MinMax3/5
  CAN Unpack1/6 -> MinMax3/6
  CAN Unpack1/7 -> MinMax3/7
  CAN Unpack1/8 -> MinMax3/8
  CAN Unpack2/1 -> MinMax2/1
  CAN Unpack2/2 -> MinMax2/2
  CAN Unpack2/3 -> MinMax2/3
  CAN Unpack2/4 -> MinMax2/4
  CAN Unpack2/5 -> MinMax2/5
  CAN Unpack2/6 -> MinMax2/6
  CAN Unpack2/7 -> MinMax2/7
  CAN Unpack2/8 -> MinMax2/8
  CAN Unpack3/1 -> MinMax/1
  CAN Unpack3/2 -> MinMax/2
  CAN Unpack3/3 -> MinMax/3
  CAN Unpack3/4 -> MinMax/4
  CAN Unpack3/5 -> MinMax/5
  CAN Unpack3/6 -> MinMax/6
  CAN Unpack3/7 -> MinMax/7
  CAN Unpack3/8 -> MinMax/8
  CAN Unpack4/1 -> MinMax1/1
  CAN Unpack4/2 -> MinMax1/2
  CAN Unpack4/3 -> MinMax1/3
  CAN Unpack4/4 -> MinMax1/4
  CAN Unpack4/5 -> MinMax1/5
  CAN Unpack4/6 -> MinMax1/6
  CAN Unpack4/7 -> MinMax1/7
  CAN Unpack4/8 -> MinMax1/8
  CAN Unpack5/1 -> MinMax5/1
  CAN Unpack5/2 -> MinMax5/2
  CAN Unpack5/3 -> MinMax5/3
  CAN Unpack5/4 -> MinMax5/4
  CAN Unpack5/5 -> MinMax5/5
  CAN Unpack5/6 -> MinMax5/6
  CAN Unpack5/7 -> MinMax5/7
  CAN Unpack5/8 -> MinMax5/8

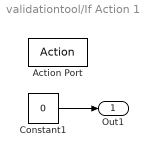
== system validationtool/If Action 1 ==
  Action Port : ActionPort  ActionPortLabel=if(u1 == 0)
  Constant1 : Constant  Value=0  OutDataTypeStr=double  SampleTime=1
  Out1 : Outport
  wires:
  Constant1/1 -> Out1/1

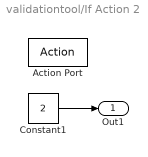
== system validationtool/If Action 2 ==
  Action Port : ActionPort  ActionPortLabel=else
  Constant1 : Constant  Value=2  OutDataTypeStr=double  SampleTime=1
  Out1 : Outport
  wires:
  Constant1/1 -> Out1/1

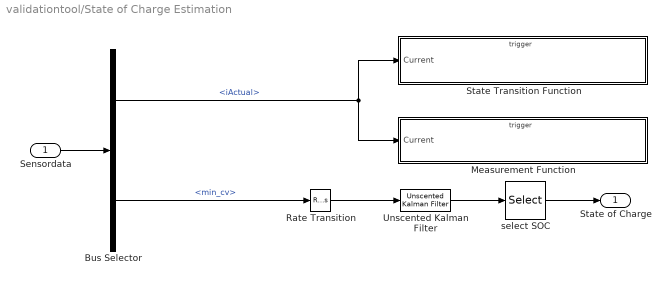
== system validationtool/State of Charge Estimation ==
  Sensordata : Inport
  Bus Selector : BusSelector  OutputSignals=iActual,min_cv
  Measurement Function : Subsystem  TreatAsAtomicUnit=on
  Rate Transition : RateTransition
  State Transition Function : Subsystem  TreatAsAtomicUnit=on
  Unscented Kalman Filter : sharedTrackingLibrary/Unscented Kalman Filter  StateTransitionFcn=StateFcn  HasAdditiveProcessNoise=Additive  ProcessNoise=1e-10*eye(3)  HasTimeVaryingProcessNoise=off  HasStateTransitionFcnExtraArgument=0  InitialState=[0.95; 0; 0]  InitialStateCovariance=[1e-2 1 1]  Alpha=1  Beta=2  Kappa=0  MeasurementFcn1=MeasurementFcn  HasMeasurementEnablePort1=off  HasAdditiveMeasurementNoise1=Additive  MeasurementNoise1=0.5  HasTimeVaryingMeasurementNoise1=off  HasMeasurementFcnExtraArgument1=0  MeasurementFcn2=myMeasurementFcn  HasMeasurementEnablePort2=off  HasAdditiveMeasurementNoise2=Additive  MeasurementNoise2=1  HasTimeVaryingMeasurementNoise2=off  HasMeasurementFcnExtraArgument2=0  MeasurementFcn3=myMeasurementFcn  HasMeasurementEnablePort3=off  HasAdditiveMeasurementNoise3=Additive  MeasurementNoise3=1  HasTimeVaryingMeasurementNoise3=off  HasMeasurementFcnExtraArgument3=0  MeasurementFcn4=myMeasurementFcn  HasMeasurementEnablePort4=off  HasAdditiveMeasurementNoise4=Additive  MeasurementNoise4=1  HasTimeVaryingMeasurementNoise4=off  HasMeasurementFcnExtraArgument4=0  MeasurementFcn5=myMeasurementFcn  HasMeasurementEnablePort5=off  HasAdditiveMeasurementNoise5=Additive  MeasurementNoise5=1  HasTimeVaryingMeasurementNoise5=off  HasMeasurementFcnExtraArgument5=0  EnableMultirate=off  StateTransitionFcnSampleTime=-1  MeasurementFcn1SampleTime=-1  MeasurementFcn2SampleTime=-1  MeasurementFcn3SampleTime=-1  MeasurementFcn4SampleTime=-1  MeasurementFcn5SampleTime=-1  UseCurrentEstimator=on  OutputStateCovariance=off  DataType=double  SampleTime=Ts  NumberOfMeasurements=1
      settings: SourceProductBaseCode=CT
  select SOC : Selector  InputPortWidth=3  IndexOptions=Index vector (dialog)  Indices=1  OutputSizes=1
  State of Charge : Outport
  wires:
  Sensordata/1 -> Bus Selector/1
  Bus Selector/2 -> Rate Transition/1  "<min_cv>"
  Bus Selector/1 -> State Transition Function/1(Current), Measurement Function/1(Current)  "<iActual>"
  Unscented Kalman Filter/1 -> select SOC/1
  Rate Transition/1 -> Unscented Kalman Filter/1
  select SOC/1 -> State of Charge/1

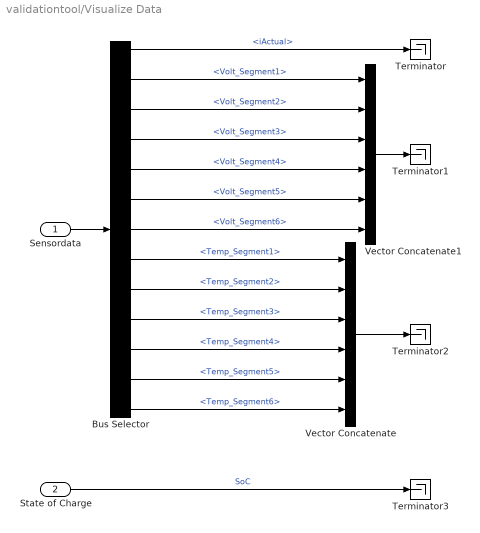
== system validationtool/Visualize Data ==
  Sensordata : Inport
  State of Charge : Inport  Port=2
  Bus Selector : BusSelector  OutputSignals=iActual,Volt_Segment1,Volt_Segment2,Volt_Segment3,Volt_Segment4,Volt_Segment5,Volt_Segment6,Temp_Segment1,Temp_Segment2,Temp_Segment3,Temp_Segment4,Temp_Segment5,Temp_Segment6
  Terminator{,1..3} (4 alike) : Terminator
  Vector Concatenate : Concatenate  NumInputs=6
  Vector Concatenate1 : Concatenate  NumInputs=6
  wires:
  Sensordata/1 -> Bus Selector/1
  Bus Selector/8 -> Vector Concatenate/1  "<Temp_Segment1>"
  Bus Selector/9 -> Vector Concatenate/2  "<Temp_Segment2>"
  Bus Selector/10 -> Vector Concatenate/3  "<Temp_Segment3>"
  Bus Selector/11 -> Vector Concatenate/4  "<Temp_Segment4>"
  Bus Selector/12 -> Vector Concatenate/5  "<Temp_Segment5>"
  Bus Selector/13 -> Vector Concatenate/6  "<Temp_Segment6>"
  Vector Concatenate/1 -> Terminator2/1
  Bus Selector/2 -> Vector Concatenate1/1  "<Volt_Segment1>"
  Bus Selector/3 -> Vector Concatenate1/2  "<Volt_Segment2>"
  Bus Selector/4 -> Vector Concatenate1/3  "<Volt_Segment3>"
  Bus Selector/5 -> Vector Concatenate1/4  "<Volt_Segment4>"
  Bus Selector/6 -> Vector Concatenate1/5  "<Volt_Segment5>"
  Bus Selector/7 -> Vector Concatenate1/6  "<Volt_Segment6>"
  Vector Concatenate1/1 -> Terminator1/1
  Bus Selector/1 -> Terminator/1  "<iActual>"
  State of Charge/1 -> Terminator3/1  "SoC"

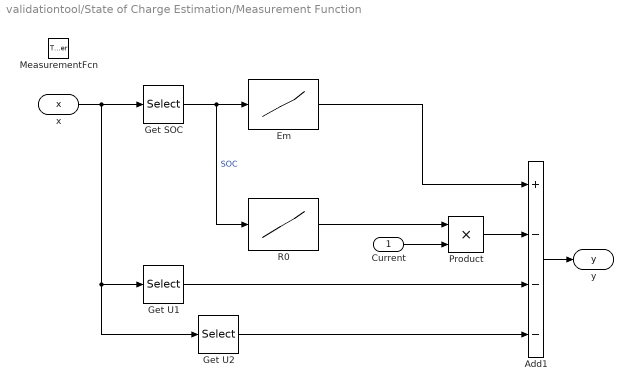
== system validationtool/State of Charge Estimation/Measurement Function ==
  Current : Inport
  MeasurementFcn : TriggerPort  TriggerType=function-call  IsSimulinkFunction=on  FunctionName=MeasurementFcn  VariantControl=Variant
  Add1 : Sum  Inputs=+---
  Em : Lookup_n-D  NumberOfTableDimensions=1  BreakpointsForDimension1=Battery.SOC_LUT  BreakpointsForDimension2=Battery.Temperature_LUT  Table=Battery.Em_LUT  InternalRulePriority=Speed  RndMeth=Simplest  InputSameDT=on
  Get SOC : Selector  InputPortWidth=3  IndexOptions=Index vector (dialog)  Indices=[1]  OutputSizes=1
  Get U1 : Selector  InputPortWidth=3  IndexOptions=Index vector (dialog)  Indices=2  OutputSizes=1
  Get U2 : Selector  InputPortWidth=3  IndexOptions=Index vector (dialog)  Indices=3  OutputSizes=1
  Product : Product
  "R0 " : Lookup_n-D  NumberOfTableDimensions=1  BreakpointsForDimension1=Battery.SOC_LUT  BreakpointsForDimension2=Battery.Temperature_LUT  Table=Battery.R0_LUT  InternalRulePriority=Speed  RndMeth=Simplest  InputSameDT=on
  x : ArgIn  DisableCoverage=on  PortDimensions=3  ArgumentName=x
  y : ArgOut  DisableCoverage=on  ArgumentName=y
  wires:
  x/1 -> Get U2/1, Get U1/1, Get SOC/1
  Get SOC/1 -> Em/1, "R0 "/1  "SOC"
  Em/1 -> Add1/1
  Add1/1 -> y/1
  "R0 "/1 -> Product/1
  Current/1 -> Product/2
  Product/1 -> Add1/2
  Get U1/1 -> Add1/3
  Get U2/1 -> Add1/4

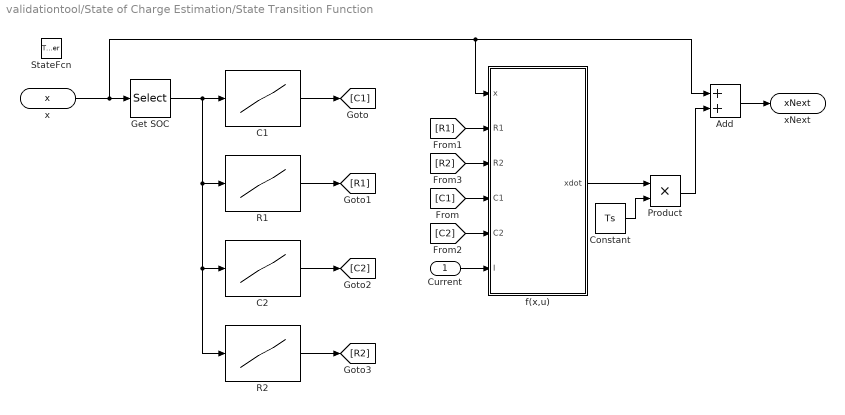
== system validationtool/State of Charge Estimation/State Transition Function ==
  Current : Inport
  StateFcn : TriggerPort  TriggerType=function-call  IsSimulinkFunction=on  FunctionName=StateFcn  VariantControl=Variant
  Add : Sum
  C1 : Lookup_n-D  NumberOfTableDimensions=1  BreakpointsForDimension1=Battery.SOC_LUT  BreakpointsForDimension2=Battery.Temperature_LUT  Table=Battery.C1_LUT  InternalRulePriority=Speed  RndMeth=Simplest  InputSameDT=on
  C2 : Lookup_n-D  NumberOfTableDimensions=1  BreakpointsForDimension1=Battery.SOC_LUT  BreakpointsForDimension2=Battery.Temperature_LUT  Table=Battery.C2_LUT  InternalRulePriority=Speed  RndMeth=Simplest  InputSameDT=on
  Constant : Constant  Value=Ts
  Get SOC : Selector  InputPortWidth=3  IndexOptions=Index vector (dialog)  Indices=1  OutputSizes=1
  Product : Product
  R1 : Lookup_n-D  NumberOfTableDimensions=1  BreakpointsForDimension1=Battery.SOC_LUT  BreakpointsForDimension2=Battery.Temperature_LUT  Table=Battery.R1_LUT  InternalRulePriority=Speed  RndMeth=Simplest  InputSameDT=on
  R2 : Lookup_n-D  NumberOfTableDimensions=1  BreakpointsForDimension1=Battery.SOC_LUT  BreakpointsForDimension2=Battery.Temperature_LUT  Table=Battery.R2_LUT  InternalRulePriority=Speed  RndMeth=Simplest  InputSameDT=on
  f(x,u) : MATLAB Function  TreatAsAtomicUnit=on
  x : ArgIn  DisableCoverage=on  PortDimensions=3  ArgumentName=x
  xNext : ArgOut  DisableCoverage=on  PortDimensions=3  ArgumentName=xNext
  wires:
  x/1 -> f(x,u)/1(x), Add/1, Get SOC/1
  Add/1 -> xNext/1
  Get SOC/1 -> R2/1, C2/1, R1/1, C1/1
  Constant/1 -> Product/2
  f(x,u)/1(xdot) -> Product/1
  Product/1 -> Add/2
  C1/1 -> [C1]
  [C1] -> f(x,u)/4(C1)
  R1/1 -> [R1]
  [R1] -> f(x,u)/2(R1)
  C2/1 -> [C2]
  [C2] -> f(x,u)/5(C2)
  R2/1 -> [R2]
  [R2] -> f(x,u)/3(R2)
  Current/1 -> f(x,u)/6(I)

== matlab function validationtool/State of Charge Estimation/State Transition Function/f(x,u) ==
  data: x input; R1 input; R2 input; C1 input; C2 input; I input; xdot output
function xdot = fx(x,R1,R2,C1,C2,I)
xdot = zeros(size(x));
U1 = x(2);
U2 = x(3);
xdot(2) = -1/C1*U1 + I/(C1/R1);
xdot(3) = -1/C2*U2 + I/(C2/R2);
